simulink model "canrx_0x586"  (R2022b)
settings: Solver=VariableStepAuto  StartTime=0.0  StopTime=10.0  RelTol=1e-3
values from neighbouring files (symbols this model uses):
  K_CAN_GMLAN_RX_INVALID_SELECT = 0.0    [canrx_0x586.sldd]
  PLCANC_APCNTL_RQST_SEL_GMLAN = 1.0    [canrx_0x586.sldd]
  PLCANC_APCNTL_RQST_SEL_J1939 = 0.0    [canrx_0x586.sldd]
undefined symbols (not defined in the file or in its folder): K_CAN_GMLAN_RX_DEFAULT_GPS_ALTITUDE, K_CAN_GMLAN_RX_DEFAULT_GPS_ANTENNA_STAT, K_CAN_GMLAN_RX_DEFAULT_GPS_DIRECTION, K_CAN_GMLAN_RX_DEFAULT_GPS_HDOP, K_CAN_GMLAN_RX_DEFAULT_GPS_LATITUDE, K_CAN_GMLAN_RX_DEFAULT_GPS_LONGITUDE, K_CAN_GMLAN_RX_DEFAULT_GPS_SG_UB, K_CAN_GMLAN_RX_DEFAULT_GPS_TIME, K_CAN_GMLAN_RX_DEFAULT_GPS_VEH_SPEED, K_CAN_RQST_SEL_1, K_CAN_RQST_SEL_2, K_CAN_RX_SEL_2, K_RQST_DRCT_2
libraries: simulink x9
(part 1 of 2)
settings Model: DataDictionary=canrx_0x586.sldd  Creator=Castiel  LastModifiedBy=Castiel

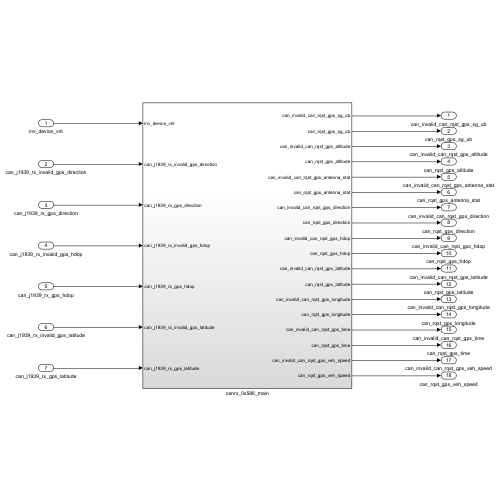
[thumbnail: Simulink's stored preview of the top-level diagram]
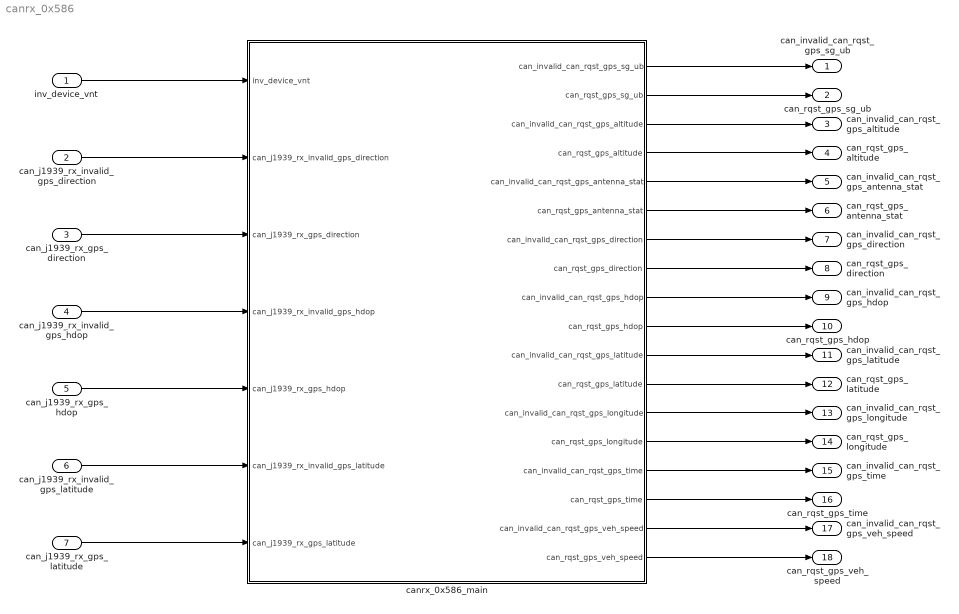
== system canrx_0x586 ==
  inv_device_vnt : Inport
  can_j1939_rx_invalid_gps_direction : Inport  Port=2
  can_j1939_rx_gps_direction : Inport  Port=3
  can_j1939_rx_invalid_gps_hdop : Inport  Port=4
  can_j1939_rx_gps_hdop : Inport  Port=5
  can_j1939_rx_invalid_gps_latitude : Inport  Port=6
  can_j1939_rx_gps_latitude : Inport  Port=7
  canrx_0x586_main : Subsystem
  can_invalid_can_rqst_gps_sg_ub : Outport
  can_rqst_gps_sg_ub : Outport  Port=2
  can_invalid_can_rqst_gps_altitude : Outport  Port=3
  can_rqst_gps_altitude : Outport  Port=4
  can_invalid_can_rqst_gps_antenna_stat : Outport  Port=5
  can_rqst_gps_antenna_stat : Outport  Port=6
  can_invalid_can_rqst_gps_direction : Outport  Port=7
  can_rqst_gps_direction : Outport  Port=8
  can_invalid_can_rqst_gps_hdop : Outport  Port=9
  can_rqst_gps_hdop : Outport  Port=10
  can_invalid_can_rqst_gps_latitude : Outport  Port=11
  can_rqst_gps_latitude : Outport  Port=12
  can_invalid_can_rqst_gps_longitude : Outport  Port=13
  can_rqst_gps_longitude : Outport  Port=14
  can_invalid_can_rqst_gps_time : Outport  Port=15
  can_rqst_gps_time : Outport  Port=16
  can_invalid_can_rqst_gps_veh_speed : Outport  Port=17
  can_rqst_gps_veh_speed : Outport  Port=18
  wires:
  inv_device_vnt/1 -> canrx_0x586_main/1(inv_device_vnt)
  can_j1939_rx_invalid_gps_direction/1 -> canrx_0x586_main/2(can_j1939_rx_invalid_gps_direction)
  can_j1939_rx_gps_direction/1 -> canrx_0x586_main/3(can_j1939_rx_gps_direction)
  can_j1939_rx_invalid_gps_hdop/1 -> canrx_0x586_main/4(can_j1939_rx_invalid_gps_hdop)
  can_j1939_rx_gps_hdop/1 -> canrx_0x586_main/5(can_j1939_rx_gps_hdop)
  can_j1939_rx_invalid_gps_latitude/1 -> canrx_0x586_main/6(can_j1939_rx_invalid_gps_latitude)
  can_j1939_rx_gps_latitude/1 -> canrx_0x586_main/7(can_j1939_rx_gps_latitude)
  canrx_0x586_main/1(can_invalid_can_rqst_gps_sg_ub) -> can_invalid_can_rqst_gps_sg_ub/1
  canrx_0x586_main/2(can_rqst_gps_sg_ub) -> can_rqst_gps_sg_ub/1
  canrx_0x586_main/3(can_invalid_can_rqst_gps_altitude) -> can_invalid_can_rqst_gps_altitude/1
  canrx_0x586_main/4(can_rqst_gps_altitude) -> can_rqst_gps_altitude/1
  canrx_0x586_main/5(can_invalid_can_rqst_gps_antenna_stat) -> can_invalid_can_rqst_gps_antenna_stat/1
  canrx_0x586_main/6(can_rqst_gps_antenna_stat) -> can_rqst_gps_antenna_stat/1
  canrx_0x586_main/7(can_invalid_can_rqst_gps_direction) -> can_invalid_can_rqst_gps_direction/1
  canrx_0x586_main/8(can_rqst_gps_direction) -> can_rqst_gps_direction/1
  canrx_0x586_main/9(can_invalid_can_rqst_gps_hdop) -> can_invalid_can_rqst_gps_hdop/1
  canrx_0x586_main/10(can_rqst_gps_hdop) -> can_rqst_gps_hdop/1
  canrx_0x586_main/11(can_invalid_can_rqst_gps_latitude) -> can_invalid_can_rqst_gps_latitude/1
  canrx_0x586_main/12(can_rqst_gps_latitude) -> can_rqst_gps_latitude/1
  canrx_0x586_main/13(can_invalid_can_rqst_gps_longitude) -> can_invalid_can_rqst_gps_longitude/1
  canrx_0x586_main/14(can_rqst_gps_longitude) -> can_rqst_gps_longitude/1
  canrx_0x586_main/15(can_invalid_can_rqst_gps_time) -> can_invalid_can_rqst_gps_time/1
  canrx_0x586_main/16(can_rqst_gps_time) -> can_rqst_gps_time/1
  canrx_0x586_main/17(can_invalid_can_rqst_gps_veh_speed) -> can_invalid_can_rqst_gps_veh_speed/1
  canrx_0x586_main/18(can_rqst_gps_veh_speed) -> can_rqst_gps_veh_speed/1

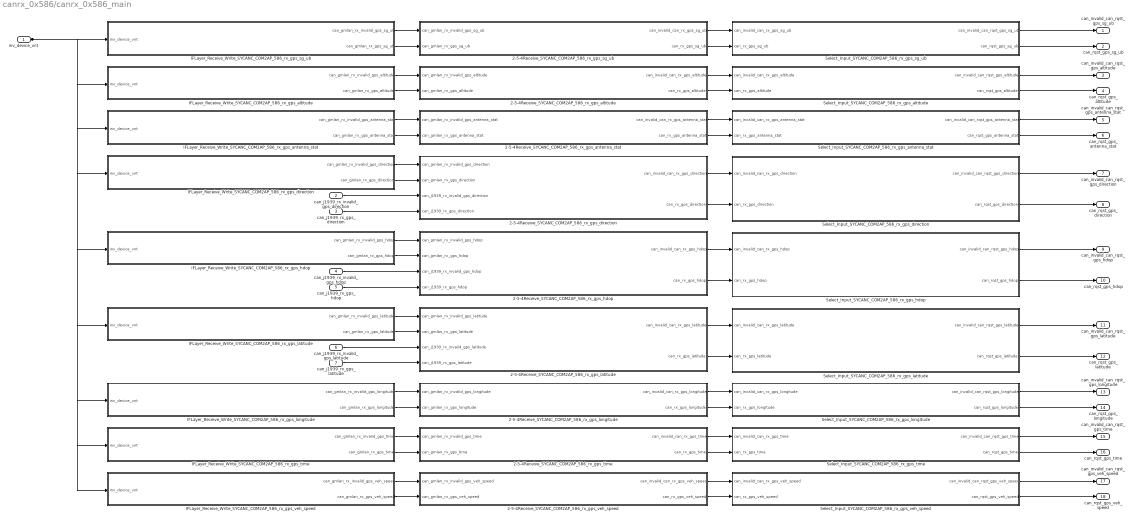
== system canrx_0x586/canrx_0x586_main ==
  inv_device_vnt : Inport
  can_j1939_rx_invalid_gps_direction : Inport  Port=2
  can_j1939_rx_gps_direction : Inport  Port=3
  can_j1939_rx_invalid_gps_hdop : Inport  Port=4
  can_j1939_rx_gps_hdop : Inport  Port=5
  can_j1939_rx_invalid_gps_latitude : Inport  Port=6
  can_j1939_rx_gps_latitude : Inport  Port=7
  2-5-4Receive_SYCANC_COM2AP_586_rx_gps_altitude : Subsystem  TreatAsAtomicUnit=on
      settings: RTWSystemCode=Nonreusable function
  2-5-4Receive_SYCANC_COM2AP_586_rx_gps_antenna_stat : Subsystem  TreatAsAtomicUnit=on
      settings: RTWSystemCode=Nonreusable function
  2-5-4Receive_SYCANC_COM2AP_586_rx_gps_direction : Subsystem  TreatAsAtomicUnit=on
      settings: RTWSystemCode=Nonreusable function
  2-5-4Receive_SYCANC_COM2AP_586_rx_gps_hdop : Subsystem  TreatAsAtomicUnit=on
      settings: RTWSystemCode=Nonreusable function
  2-5-4Receive_SYCANC_COM2AP_586_rx_gps_latitude : Subsystem  TreatAsAtomicUnit=on
      settings: RTWSystemCode=Nonreusable function
  2-5-4Receive_SYCANC_COM2AP_586_rx_gps_longitude : Subsystem  TreatAsAtomicUnit=on
      settings: RTWSystemCode=Nonreusable function
  2-5-4Receive_SYCANC_COM2AP_586_rx_gps_sg_ub : Subsystem  TreatAsAtomicUnit=on
      settings: RTWSystemCode=Nonreusable function
  2-5-4Receive_SYCANC_COM2AP_586_rx_gps_time : Subsystem  TreatAsAtomicUnit=on
      settings: RTWSystemCode=Nonreusable function
  2-5-4Receive_SYCANC_COM2AP_586_rx_gps_veh_speed : Subsystem  TreatAsAtomicUnit=on
      settings: RTWSystemCode=Nonreusable function
  IFLayer_Receive_Write_SYCANC_COM2AP_586_rx_gps_altitude : Subsystem  TreatAsAtomicUnit=on
      settings: RTWSystemCode=Nonreusable function
  IFLayer_Receive_Write_SYCANC_COM2AP_586_rx_gps_antenna_stat : Subsystem  TreatAsAtomicUnit=on
      settings: RTWSystemCode=Nonreusable function
  IFLayer_Receive_Write_SYCANC_COM2AP_586_rx_gps_direction : Subsystem  TreatAsAtomicUnit=on
      settings: RTWSystemCode=Nonreusable function
  IFLayer_Receive_Write_SYCANC_COM2AP_586_rx_gps_hdop : Subsystem  TreatAsAtomicUnit=on
      settings: RTWSystemCode=Nonreusable function
  IFLayer_Receive_Write_SYCANC_COM2AP_586_rx_gps_latitude : Subsystem  TreatAsAtomicUnit=on
      settings: RTWSystemCode=Nonreusable function
  IFLayer_Receive_Write_SYCANC_COM2AP_586_rx_gps_longitude : Subsystem  TreatAsAtomicUnit=on
      settings: RTWSystemCode=Nonreusable function
  IFLayer_Receive_Write_SYCANC_COM2AP_586_rx_gps_sg_ub : Subsystem  TreatAsAtomicUnit=on
      settings: RTWSystemCode=Nonreusable function
  IFLayer_Receive_Write_SYCANC_COM2AP_586_rx_gps_time : Subsystem  TreatAsAtomicUnit=on
      settings: RTWSystemCode=Nonreusable function
  IFLayer_Receive_Write_SYCANC_COM2AP_586_rx_gps_veh_speed : Subsystem  TreatAsAtomicUnit=on
      settings: RTWSystemCode=Nonreusable function
  Select_Input_SYCANC_COM2AP_586_rx_gps_altitude : Subsystem  TreatAsAtomicUnit=on
      settings: RTWSystemCode=Nonreusable function
  Select_Input_SYCANC_COM2AP_586_rx_gps_antenna_stat : Subsystem  TreatAsAtomicUnit=on
      settings: RTWSystemCode=Nonreusable function
  Select_Input_SYCANC_COM2AP_586_rx_gps_direction : Subsystem  TreatAsAtomicUnit=on
      settings: RTWSystemCode=Nonreusable function
  Select_Input_SYCANC_COM2AP_586_rx_gps_hdop : Subsystem  TreatAsAtomicUnit=on
      settings: RTWSystemCode=Nonreusable function
  Select_Input_SYCANC_COM2AP_586_rx_gps_latitude : Subsystem  TreatAsAtomicUnit=on
      settings: RTWSystemCode=Nonreusable function
  Select_Input_SYCANC_COM2AP_586_rx_gps_longitude : Subsystem  TreatAsAtomicUnit=on
      settings: RTWSystemCode=Nonreusable function
  Select_Input_SYCANC_COM2AP_586_rx_gps_sg_ub : Subsystem  TreatAsAtomicUnit=on
      settings: RTWSystemCode=Nonreusable function
  Select_Input_SYCANC_COM2AP_586_rx_gps_time : Subsystem  TreatAsAtomicUnit=on
      settings: RTWSystemCode=Nonreusable function
  Select_Input_SYCANC_COM2AP_586_rx_gps_veh_speed : Subsystem  TreatAsAtomicUnit=on
      settings: RTWSystemCode=Nonreusable function
  can_invalid_can_rqst_gps_sg_ub : Outport
  can_rqst_gps_sg_ub : Outport  Port=2
  can_invalid_can_rqst_gps_altitude : Outport  Port=3
  can_rqst_gps_altitude : Outport  Port=4
  can_invalid_can_rqst_gps_antenna_stat : Outport  Port=5
  can_rqst_gps_antenna_stat : Outport  Port=6
  can_invalid_can_rqst_gps_direction : Outport  Port=7
  can_rqst_gps_direction : Outport  Port=8
  can_invalid_can_rqst_gps_hdop : Outport  Port=9
  can_rqst_gps_hdop : Outport  Port=10
  can_invalid_can_rqst_gps_latitude : Outport  Port=11
  can_rqst_gps_latitude : Outport  Port=12
  can_invalid_can_rqst_gps_longitude : Outport  Port=13
  can_rqst_gps_longitude : Outport  Port=14
  can_invalid_can_rqst_gps_time : Outport  Port=15
  can_rqst_gps_time : Outport  Port=16
  can_invalid_can_rqst_gps_veh_speed : Outport  Port=17
  can_rqst_gps_veh_speed : Outport  Port=18
  wires:
  IFLayer_Receive_Write_SYCANC_COM2AP_586_rx_gps_sg_ub/2(can_gmlan_rx_gps_sg_ub) -> 2-5-4Receive_SYCANC_COM2AP_586_rx_gps_sg_ub/2(can_gmlan_rx_gps_sg_ub)
  IFLayer_Receive_Write_SYCANC_COM2AP_586_rx_gps_sg_ub/1(can_gmlan_rx_invalid_gps_sg_ub) -> 2-5-4Receive_SYCANC_COM2AP_586_rx_gps_sg_ub/1(can_gmlan_rx_invalid_gps_sg_ub)
  2-5-4Receive_SYCANC_COM2AP_586_rx_gps_sg_ub/1(can_invalid_can_rx_gps_sg_ub) -> Select_Input_SYCANC_COM2AP_586_rx_gps_sg_ub/1(can_invalid_can_rx_gps_sg_ub)
  2-5-4Receive_SYCANC_COM2AP_586_rx_gps_sg_ub/2(can_rx_gps_sg_ub) -> Select_Input_SYCANC_COM2AP_586_rx_gps_sg_ub/2(can_rx_gps_sg_ub)
  inv_device_vnt/1 -> IFLayer_Receive_Write_SYCANC_COM2AP_586_rx_gps_sg_ub/1(inv_device_vnt), IFLayer_Receive_Write_SYCANC_COM2AP_586_rx_gps_altitude/1(inv_device_vnt), IFLayer_Receive_Write_SYCANC_COM2AP_586_rx_gps_antenna_stat/1(inv_device_vnt), IFLayer_Receive_Write_SYCANC_COM2AP_586_rx_gps_direction/1(inv_device_vnt), IFLayer_Receive_Write_SYCANC_COM2AP_586_rx_gps_hdop/1(inv_device_vnt), IFLayer_Receive_Write_SYCANC_COM2AP_586_rx_gps_latitude/1(inv_device_vnt), IFLayer_Receive_Write_SYCANC_COM2AP_586_rx_gps_longitude/1(inv_device_vnt), IFLayer_Receive_Write_SYCANC_COM2AP_586_rx_gps_time/1(inv_device_vnt), IFLayer_Receive_Write_SYCANC_COM2AP_586_rx_gps_veh_speed/1(inv_device_vnt)
  Select_Input_SYCANC_COM2AP_586_rx_gps_sg_ub/1(can_invalid_can_rqst_gps_sg_ub) -> can_invalid_can_rqst_gps_sg_ub/1
  Select_Input_SYCANC_COM2AP_586_rx_gps_sg_ub/2(can_rqst_gps_sg_ub) -> can_rqst_gps_sg_ub/1
  IFLayer_Receive_Write_SYCANC_COM2AP_586_rx_gps_altitude/2(can_gmlan_rx_gps_altitude) -> 2-5-4Receive_SYCANC_COM2AP_586_rx_gps_altitude/2(can_gmlan_rx_gps_altitude)
  IFLayer_Receive_Write_SYCANC_COM2AP_586_rx_gps_altitude/1(can_gmlan_rx_invalid_gps_altitude) -> 2-5-4Receive_SYCANC_COM2AP_586_rx_gps_altitude/1(can_gmlan_rx_invalid_gps_altitude)
  2-5-4Receive_SYCANC_COM2AP_586_rx_gps_altitude/1(can_invalid_can_rx_gps_altitude) -> Select_Input_SYCANC_COM2AP_586_rx_gps_altitude/1(can_invalid_can_rx_gps_altitude)
  2-5-4Receive_SYCANC_COM2AP_586_rx_gps_altitude/2(can_rx_gps_altitude) -> Select_Input_SYCANC_COM2AP_586_rx_gps_altitude/2(can_rx_gps_altitude)
  Select_Input_SYCANC_COM2AP_586_rx_gps_altitude/1(can_invalid_can_rqst_gps_altitude) -> can_invalid_can_rqst_gps_altitude/1
  Select_Input_SYCANC_COM2AP_586_rx_gps_altitude/2(can_rqst_gps_altitude) -> can_rqst_gps_altitude/1
  IFLayer_Receive_Write_SYCANC_COM2AP_586_rx_gps_antenna_stat/2(can_gmlan_rx_gps_antenna_stat) -> 2-5-4Receive_SYCANC_COM2AP_586_rx_gps_antenna_stat/2(can_gmlan_rx_gps_antenna_stat)
  IFLayer_Receive_Write_SYCANC_COM2AP_586_rx_gps_antenna_stat/1(can_gmlan_rx_invalid_gps_antenna_stat) -> 2-5-4Receive_SYCANC_COM2AP_586_rx_gps_antenna_stat/1(can_gmlan_rx_invalid_gps_antenna_stat)
  2-5-4Receive_SYCANC_COM2AP_586_rx_gps_antenna_stat/1(can_invalid_can_rx_gps_antenna_stat) -> Select_Input_SYCANC_COM2AP_586_rx_gps_antenna_stat/1(can_invalid_can_rx_gps_antenna_stat)
  2-5-4Receive_SYCANC_COM2AP_586_rx_gps_antenna_stat/2(can_rx_gps_antenna_stat) -> Select_Input_SYCANC_COM2AP_586_rx_gps_antenna_stat/2(can_rx_gps_antenna_stat)
  Select_Input_SYCANC_COM2AP_586_rx_gps_antenna_stat/1(can_invalid_can_rqst_gps_antenna_stat) -> can_invalid_can_rqst_gps_antenna_stat/1
  Select_Input_SYCANC_COM2AP_586_rx_gps_antenna_stat/2(can_rqst_gps_antenna_stat) -> can_rqst_gps_antenna_stat/1
  IFLayer_Receive_Write_SYCANC_COM2AP_586_rx_gps_direction/2(can_gmlan_rx_gps_direction) -> 2-5-4Receive_SYCANC_COM2AP_586_rx_gps_direction/2(can_gmlan_rx_gps_direction)
  IFLayer_Receive_Write_SYCANC_COM2AP_586_rx_gps_direction/1(can_gmlan_rx_invalid_gps_direction) -> 2-5-4Receive_SYCANC_COM2AP_586_rx_gps_direction/1(can_gmlan_rx_invalid_gps_direction)
  2-5-4Receive_SYCANC_COM2AP_586_rx_gps_direction/1(can_invalid_can_rx_gps_direction) -> Select_Input_SYCANC_COM2AP_586_rx_gps_direction/1(can_invalid_can_rx_gps_direction)
  2-5-4Receive_SYCANC_COM2AP_586_rx_gps_direction/2(can_rx_gps_direction) -> Select_Input_SYCANC_COM2AP_586_rx_gps_direction/2(can_rx_gps_direction)
  can_j1939_rx_invalid_gps_direction/1 -> 2-5-4Receive_SYCANC_COM2AP_586_rx_gps_direction/3(can_j1939_rx_invalid_gps_direction)
  can_j1939_rx_gps_direction/1 -> 2-5-4Receive_SYCANC_COM2AP_586_rx_gps_direction/4(can_j1939_rx_gps_direction)
  Select_Input_SYCANC_COM2AP_586_rx_gps_direction/1(can_invalid_can_rqst_gps_direction) -> can_invalid_can_rqst_gps_direction/1
  Select_Input_SYCANC_COM2AP_586_rx_gps_direction/2(can_rqst_gps_direction) -> can_rqst_gps_direction/1
  IFLayer_Receive_Write_SYCANC_COM2AP_586_rx_gps_hdop/2(can_gmlan_rx_gps_hdop) -> 2-5-4Receive_SYCANC_COM2AP_586_rx_gps_hdop/2(can_gmlan_rx_gps_hdop)
  IFLayer_Receive_Write_SYCANC_COM2AP_586_rx_gps_hdop/1(can_gmlan_rx_invalid_gps_hdop) -> 2-5-4Receive_SYCANC_COM2AP_586_rx_gps_hdop/1(can_gmlan_rx_invalid_gps_hdop)
  2-5-4Receive_SYCANC_COM2AP_586_rx_gps_hdop/1(can_invalid_can_rx_gps_hdop) -> Select_Input_SYCANC_COM2AP_586_rx_gps_hdop/1(can_invalid_can_rx_gps_hdop)
  2-5-4Receive_SYCANC_COM2AP_586_rx_gps_hdop/2(can_rx_gps_hdop) -> Select_Input_SYCANC_COM2AP_586_rx_gps_hdop/2(can_rx_gps_hdop)
  can_j1939_rx_invalid_gps_hdop/1 -> 2-5-4Receive_SYCANC_COM2AP_586_rx_gps_hdop/3(can_j1939_rx_invalid_gps_hdop)
  can_j1939_rx_gps_hdop/1 -> 2-5-4Receive_SYCANC_COM2AP_586_rx_gps_hdop/4(can_j1939_rx_gps_hdop)
  Select_Input_SYCANC_COM2AP_586_rx_gps_hdop/1(can_invalid_can_rqst_gps_hdop) -> can_invalid_can_rqst_gps_hdop/1
  Select_Input_SYCANC_COM2AP_586_rx_gps_hdop/2(can_rqst_gps_hdop) -> can_rqst_gps_hdop/1
  IFLayer_Receive_Write_SYCANC_COM2AP_586_rx_gps_latitude/2(can_gmlan_rx_gps_latitude) -> 2-5-4Receive_SYCANC_COM2AP_586_rx_gps_latitude/2(can_gmlan_rx_gps_latitude)
  IFLayer_Receive_Write_SYCANC_COM2AP_586_rx_gps_latitude/1(can_gmlan_rx_invalid_gps_latitude) -> 2-5-4Receive_SYCANC_COM2AP_586_rx_gps_latitude/1(can_gmlan_rx_invalid_gps_latitude)
  2-5-4Receive_SYCANC_COM2AP_586_rx_gps_latitude/1(can_invalid_can_rx_gps_latitude) -> Select_Input_SYCANC_COM2AP_586_rx_gps_latitude/1(can_invalid_can_rx_gps_latitude)
  2-5-4Receive_SYCANC_COM2AP_586_rx_gps_latitude/2(can_rx_gps_latitude) -> Select_Input_SYCANC_COM2AP_586_rx_gps_latitude/2(can_rx_gps_latitude)
  can_j1939_rx_invalid_gps_latitude/1 -> 2-5-4Receive_SYCANC_COM2AP_586_rx_gps_latitude/3(can_j1939_rx_invalid_gps_latitude)
  can_j1939_rx_gps_latitude/1 -> 2-5-4Receive_SYCANC_COM2AP_586_rx_gps_latitude/4(can_j1939_rx_gps_latitude)
  Select_Input_SYCANC_COM2AP_586_rx_gps_latitude/1(can_invalid_can_rqst_gps_latitude) -> can_invalid_can_rqst_gps_latitude/1
  Select_Input_SYCANC_COM2AP_586_rx_gps_latitude/2(can_rqst_gps_latitude) -> can_rqst_gps_latitude/1
  IFLayer_Receive_Write_SYCANC_COM2AP_586_rx_gps_longitude/2(can_gmlan_rx_gps_longitude) -> 2-5-4Receive_SYCANC_COM2AP_586_rx_gps_longitude/2(can_gmlan_rx_gps_longitude)
  IFLayer_Receive_Write_SYCANC_COM2AP_586_rx_gps_longitude/1(can_gmlan_rx_invalid_gps_longitude) -> 2-5-4Receive_SYCANC_COM2AP_586_rx_gps_longitude/1(can_gmlan_rx_invalid_gps_longitude)
  2-5-4Receive_SYCANC_COM2AP_586_rx_gps_longitude/1(can_invalid_can_rx_gps_longitude) -> Select_Input_SYCANC_COM2AP_586_rx_gps_longitude/1(can_invalid_can_rx_gps_longitude)
  2-5-4Receive_SYCANC_COM2AP_586_rx_gps_longitude/2(can_rx_gps_longitude) -> Select_Input_SYCANC_COM2AP_586_rx_gps_longitude/2(can_rx_gps_longitude)
  Select_Input_SYCANC_COM2AP_586_rx_gps_longitude/1(can_invalid_can_rqst_gps_longitude) -> can_invalid_can_rqst_gps_longitude/1
  Select_Input_SYCANC_COM2AP_586_rx_gps_longitude/2(can_rqst_gps_longitude) -> can_rqst_gps_longitude/1
  IFLayer_Receive_Write_SYCANC_COM2AP_586_rx_gps_time/2(can_gmlan_rx_gps_time) -> 2-5-4Receive_SYCANC_COM2AP_586_rx_gps_time/2(can_gmlan_rx_gps_time)
  IFLayer_Receive_Write_SYCANC_COM2AP_586_rx_gps_time/1(can_gmlan_rx_invalid_gps_time) -> 2-5-4Receive_SYCANC_COM2AP_586_rx_gps_time/1(can_gmlan_rx_invalid_gps_time)
  2-5-4Receive_SYCANC_COM2AP_586_rx_gps_time/1(can_invalid_can_rx_gps_time) -> Select_Input_SYCANC_COM2AP_586_rx_gps_time/1(can_invalid_can_rx_gps_time)
  2-5-4Receive_SYCANC_COM2AP_586_rx_gps_time/2(can_rx_gps_time) -> Select_Input_SYCANC_COM2AP_586_rx_gps_time/2(can_rx_gps_time)
  Select_Input_SYCANC_COM2AP_586_rx_gps_time/1(can_invalid_can_rqst_gps_time) -> can_invalid_can_rqst_gps_time/1
  Select_Input_SYCANC_COM2AP_586_rx_gps_time/2(can_rqst_gps_time) -> can_rqst_gps_time/1
  IFLayer_Receive_Write_SYCANC_COM2AP_586_rx_gps_veh_speed/2(can_gmlan_rx_gps_veh_speed) -> 2-5-4Receive_SYCANC_COM2AP_586_rx_gps_veh_speed/2(can_gmlan_rx_gps_veh_speed)
  IFLayer_Receive_Write_SYCANC_COM2AP_586_rx_gps_veh_speed/1(can_gmlan_rx_invalid_gps_veh_speed) -> 2-5-4Receive_SYCANC_COM2AP_586_rx_gps_veh_speed/1(can_gmlan_rx_invalid_gps_veh_speed)
  2-5-4Receive_SYCANC_COM2AP_586_rx_gps_veh_speed/1(can_invalid_can_rx_gps_veh_speed) -> Select_Input_SYCANC_COM2AP_586_rx_gps_veh_speed/1(can_invalid_can_rx_gps_veh_speed)
  2-5-4Receive_SYCANC_COM2AP_586_rx_gps_veh_speed/2(can_rx_gps_veh_speed) -> Select_Input_SYCANC_COM2AP_586_rx_gps_veh_speed/2(can_rx_gps_veh_speed)
  Select_Input_SYCANC_COM2AP_586_rx_gps_veh_speed/1(can_invalid_can_rqst_gps_veh_speed) -> can_invalid_can_rqst_gps_veh_speed/1
  Select_Input_SYCANC_COM2AP_586_rx_gps_veh_speed/2(can_rqst_gps_veh_speed) -> can_rqst_gps_veh_speed/1

== system canrx_0x586/canrx_0x586_main/2-5-4Receive_SYCANC_COM2AP_586_rx_gps_altitude ==
  can_gmlan_rx_invalid_gps_altitude : Inport
  can_gmlan_rx_gps_altitude : Inport  Port=2
  can_invalid_can_rx_gps_altitude : Outport
  can_rx_gps_altitude : Outport  Port=2
  wires:
  can_gmlan_rx_gps_altitude/1 -> can_rx_gps_altitude/1
  can_gmlan_rx_invalid_gps_altitude/1 -> can_invalid_can_rx_gps_altitude/1

== system canrx_0x586/canrx_0x586_main/2-5-4Receive_SYCANC_COM2AP_586_rx_gps_antenna_stat ==
  can_gmlan_rx_invalid_gps_antenna_stat : Inport
  can_gmlan_rx_gps_antenna_stat : Inport  Port=2
  can_invalid_can_rx_gps_antenna_stat : Outport
  can_rx_gps_antenna_stat : Outport  Port=2
  wires:
  can_gmlan_rx_gps_antenna_stat/1 -> can_rx_gps_antenna_stat/1
  can_gmlan_rx_invalid_gps_antenna_stat/1 -> can_invalid_can_rx_gps_antenna_stat/1

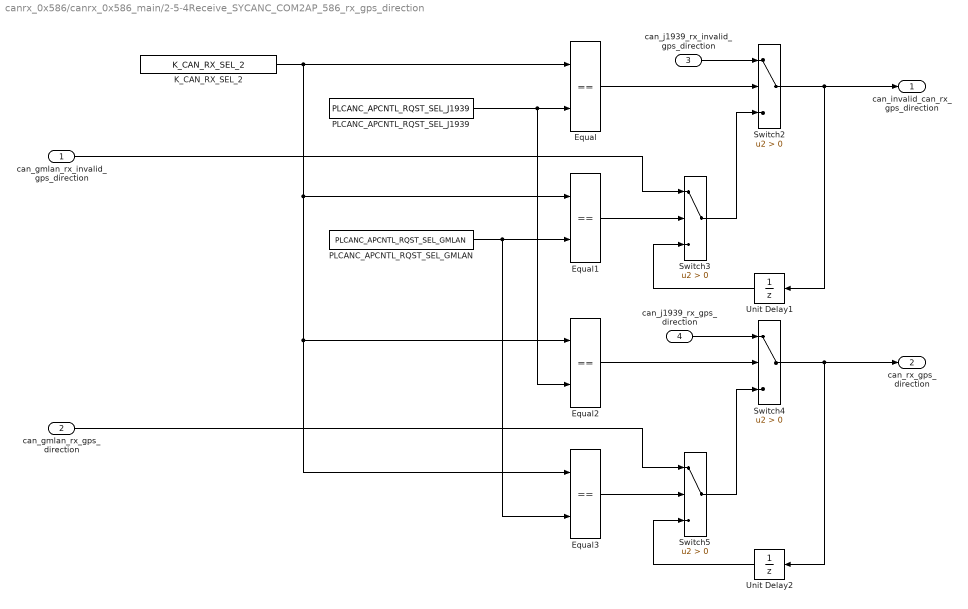
== system canrx_0x586/canrx_0x586_main/2-5-4Receive_SYCANC_COM2AP_586_rx_gps_direction ==
  can_gmlan_rx_invalid_gps_direction : Inport
  can_gmlan_rx_gps_direction : Inport  Port=2
  can_j1939_rx_invalid_gps_direction : Inport  Port=3
  can_j1939_rx_gps_direction : Inport  Port=4
  Equal{,1..3} (4 alike) : RelationalOperator  Operator===  OutDataTypeStr=boolean  RndMeth=Simplest  InputSameDT=off
  K_CAN_RX_SEL_2 : Constant  Value=K_CAN_RX_SEL_2
  PLCANC_APCNTL_RQST_SEL_GMLAN : Constant  Value=PLCANC_APCNTL_RQST_SEL_GMLAN
  PLCANC_APCNTL_RQST_SEL_J1939 : Constant  Value=PLCANC_APCNTL_RQST_SEL_J1939
  Switch{2..5} (4 alike) : Switch  Criteria=u2 > Threshold  SaturateOnIntegerOverflow=off  InputSameDT=off
  Unit Delay1 : UnitDelay  SampleTime=-1  HasFrameUpgradeWarning=on
  Unit Delay2 : UnitDelay  SampleTime=-1  HasFrameUpgradeWarning=on
  can_invalid_can_rx_gps_direction : Outport
  can_rx_gps_direction : Outport  Port=2
  wires:
  Switch3/1 -> Switch2/3
  can_j1939_rx_gps_direction/1 -> Switch4/1
  K_CAN_RX_SEL_2/1 -> Equal/1, Equal1/1, Equal2/1, Equal3/1
  Switch4/1 -> can_rx_gps_direction/1, Unit Delay2/1
  PLCANC_APCNTL_RQST_SEL_J1939/1 -> Equal/2, Equal2/2
  can_gmlan_rx_gps_direction/1 -> Switch5/1
  Equal2/1 -> Switch4/2
  can_j1939_rx_invalid_gps_direction/1 -> Switch2/1
  PLCANC_APCNTL_RQST_SEL_GMLAN/1 -> Equal1/2, Equal3/2
  can_gmlan_rx_invalid_gps_direction/1 -> Switch3/1
  Switch5/1 -> Switch4/3
  Equal3/1 -> Switch5/2
  Equal1/1 -> Switch3/2
  Unit Delay2/1 -> Switch5/3
  Switch2/1 -> can_invalid_can_rx_gps_direction/1, Unit Delay1/1
  Unit Delay1/1 -> Switch3/3
  Equal/1 -> Switch2/2

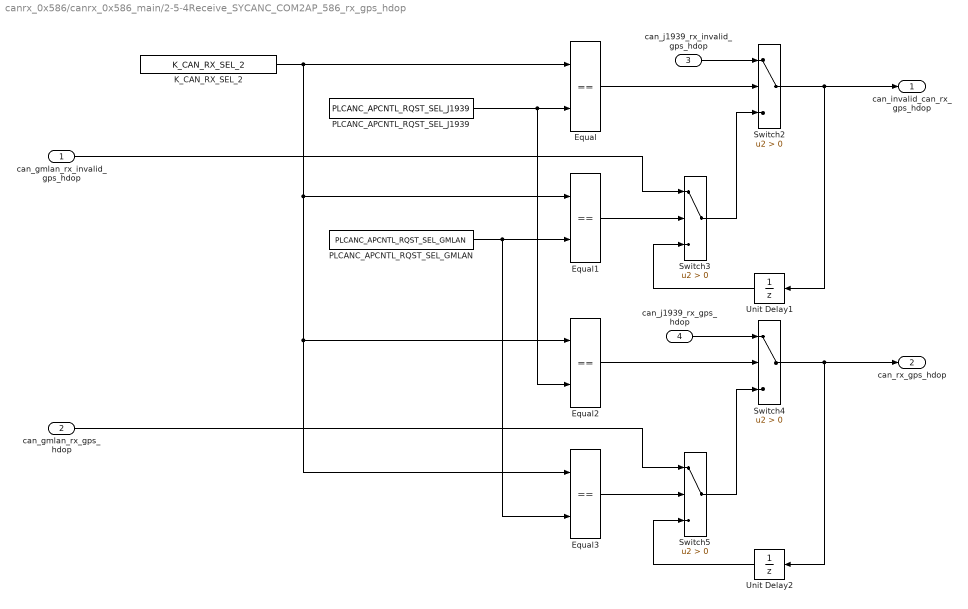
== system canrx_0x586/canrx_0x586_main/2-5-4Receive_SYCANC_COM2AP_586_rx_gps_hdop ==
  can_gmlan_rx_invalid_gps_hdop : Inport
  can_gmlan_rx_gps_hdop : Inport  Port=2
  can_j1939_rx_invalid_gps_hdop : Inport  Port=3
  can_j1939_rx_gps_hdop : Inport  Port=4
  Equal{,1..3} (4 alike) : RelationalOperator  Operator===  OutDataTypeStr=boolean  RndMeth=Simplest  InputSameDT=off
  K_CAN_RX_SEL_2 : Constant  Value=K_CAN_RX_SEL_2
  PLCANC_APCNTL_RQST_SEL_GMLAN : Constant  Value=PLCANC_APCNTL_RQST_SEL_GMLAN
  PLCANC_APCNTL_RQST_SEL_J1939 : Constant  Value=PLCANC_APCNTL_RQST_SEL_J1939
  Switch{2..5} (4 alike) : Switch  Criteria=u2 > Threshold  SaturateOnIntegerOverflow=off  InputSameDT=off
  Unit Delay1 : UnitDelay  SampleTime=-1  HasFrameUpgradeWarning=on
  Unit Delay2 : UnitDelay  SampleTime=-1  HasFrameUpgradeWarning=on
  can_invalid_can_rx_gps_hdop : Outport
  can_rx_gps_hdop : Outport  Port=2
  wires:
  Switch3/1 -> Switch2/3
  can_j1939_rx_gps_hdop/1 -> Switch4/1
  K_CAN_RX_SEL_2/1 -> Equal/1, Equal1/1, Equal2/1, Equal3/1
  Switch4/1 -> can_rx_gps_hdop/1, Unit Delay2/1
  PLCANC_APCNTL_RQST_SEL_J1939/1 -> Equal/2, Equal2/2
  can_gmlan_rx_gps_hdop/1 -> Switch5/1
  Equal2/1 -> Switch4/2
  can_j1939_rx_invalid_gps_hdop/1 -> Switch2/1
  PLCANC_APCNTL_RQST_SEL_GMLAN/1 -> Equal1/2, Equal3/2
  can_gmlan_rx_invalid_gps_hdop/1 -> Switch3/1
  Switch5/1 -> Switch4/3
  Equal3/1 -> Switch5/2
  Equal1/1 -> Switch3/2
  Unit Delay2/1 -> Switch5/3
  Switch2/1 -> can_invalid_can_rx_gps_hdop/1, Unit Delay1/1
  Unit Delay1/1 -> Switch3/3
  Equal/1 -> Switch2/2

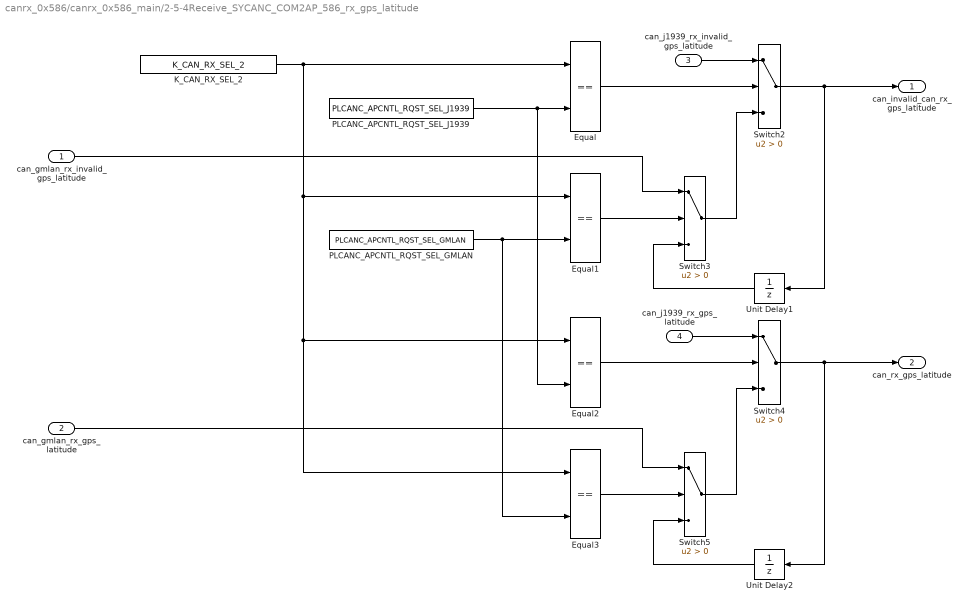
== system canrx_0x586/canrx_0x586_main/2-5-4Receive_SYCANC_COM2AP_586_rx_gps_latitude ==
  can_gmlan_rx_invalid_gps_latitude : Inport
  can_gmlan_rx_gps_latitude : Inport  Port=2
  can_j1939_rx_invalid_gps_latitude : Inport  Port=3
  can_j1939_rx_gps_latitude : Inport  Port=4
  Equal{,1..3} (4 alike) : RelationalOperator  Operator===  OutDataTypeStr=boolean  RndMeth=Simplest  InputSameDT=off
  K_CAN_RX_SEL_2 : Constant  Value=K_CAN_RX_SEL_2
  PLCANC_APCNTL_RQST_SEL_GMLAN : Constant  Value=PLCANC_APCNTL_RQST_SEL_GMLAN
  PLCANC_APCNTL_RQST_SEL_J1939 : Constant  Value=PLCANC_APCNTL_RQST_SEL_J1939
  Switch{2..5} (4 alike) : Switch  Criteria=u2 > Threshold  SaturateOnIntegerOverflow=off  InputSameDT=off
  Unit Delay1 : UnitDelay  SampleTime=-1  HasFrameUpgradeWarning=on
  Unit Delay2 : UnitDelay  SampleTime=-1  HasFrameUpgradeWarning=on
  can_invalid_can_rx_gps_latitude : Outport
  can_rx_gps_latitude : Outport  Port=2
  wires:
  Switch3/1 -> Switch2/3
  can_j1939_rx_gps_latitude/1 -> Switch4/1
  K_CAN_RX_SEL_2/1 -> Equal/1, Equal1/1, Equal2/1, Equal3/1
  Switch4/1 -> can_rx_gps_latitude/1, Unit Delay2/1
  PLCANC_APCNTL_RQST_SEL_J1939/1 -> Equal/2, Equal2/2
  can_gmlan_rx_gps_latitude/1 -> Switch5/1
  Equal2/1 -> Switch4/2
  can_j1939_rx_invalid_gps_latitude/1 -> Switch2/1
  PLCANC_APCNTL_RQST_SEL_GMLAN/1 -> Equal1/2, Equal3/2
  can_gmlan_rx_invalid_gps_latitude/1 -> Switch3/1
  Switch5/1 -> Switch4/3
  Equal3/1 -> Switch5/2
  Equal1/1 -> Switch3/2
  Unit Delay2/1 -> Switch5/3
  Switch2/1 -> can_invalid_can_rx_gps_latitude/1, Unit Delay1/1
  Unit Delay1/1 -> Switch3/3
  Equal/1 -> Switch2/2

== system canrx_0x586/canrx_0x586_main/2-5-4Receive_SYCANC_COM2AP_586_rx_gps_longitude ==
  can_gmlan_rx_invalid_gps_longitude : Inport
  can_gmlan_rx_gps_longitude : Inport  Port=2
  can_invalid_can_rx_gps_longitude : Outport
  can_rx_gps_longitude : Outport  Port=2
  wires:
  can_gmlan_rx_gps_longitude/1 -> can_rx_gps_longitude/1
  can_gmlan_rx_invalid_gps_longitude/1 -> can_invalid_can_rx_gps_longitude/1

== system canrx_0x586/canrx_0x586_main/2-5-4Receive_SYCANC_COM2AP_586_rx_gps_sg_ub ==
  can_gmlan_rx_invalid_gps_sg_ub : Inport
  can_gmlan_rx_gps_sg_ub : Inport  Port=2
  can_invalid_can_rx_gps_sg_ub : Outport
  can_rx_gps_sg_ub : Outport  Port=2
  wires:
  can_gmlan_rx_gps_sg_ub/1 -> can_rx_gps_sg_ub/1
  can_gmlan_rx_invalid_gps_sg_ub/1 -> can_invalid_can_rx_gps_sg_ub/1

== system canrx_0x586/canrx_0x586_main/2-5-4Receive_SYCANC_COM2AP_586_rx_gps_time ==
  can_gmlan_rx_invalid_gps_time : Inport
  can_gmlan_rx_gps_time : Inport  Port=2
  can_invalid_can_rx_gps_time : Outport
  can_rx_gps_time : Outport  Port=2
  wires:
  can_gmlan_rx_gps_time/1 -> can_rx_gps_time/1
  can_gmlan_rx_invalid_gps_time/1 -> can_invalid_can_rx_gps_time/1

== system canrx_0x586/canrx_0x586_main/2-5-4Receive_SYCANC_COM2AP_586_rx_gps_veh_speed ==
  can_gmlan_rx_invalid_gps_veh_speed : Inport
  can_gmlan_rx_gps_veh_speed : Inport  Port=2
  can_invalid_can_rx_gps_veh_speed : Outport
  can_rx_gps_veh_speed : Outport  Port=2
  wires:
  can_gmlan_rx_gps_veh_speed/1 -> can_rx_gps_veh_speed/1
  can_gmlan_rx_invalid_gps_veh_speed/1 -> can_invalid_can_rx_gps_veh_speed/1

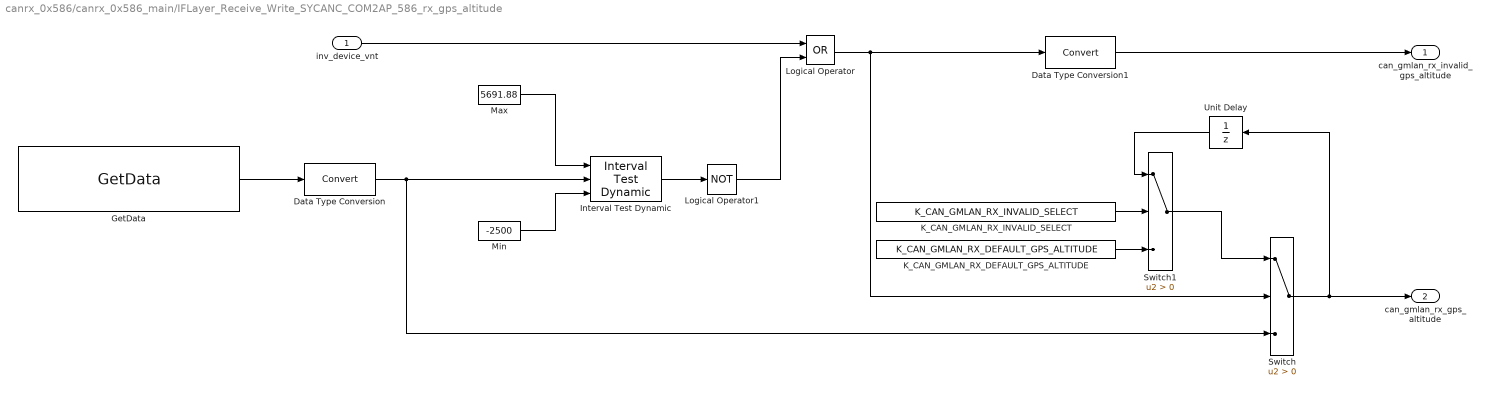
== system canrx_0x586/canrx_0x586_main/IFLayer_Receive_Write_SYCANC_COM2AP_586_rx_gps_altitude ==
  inv_device_vnt : Inport
  Data Type Conversion : DataTypeConversion  ConvertRealWorld=Stored Integer (SI)  SaturateOnIntegerOverflow=off  RndMeth=Floor
  Data Type Conversion1 : DataTypeConversion  ConvertRealWorld=Stored Integer (SI)  SaturateOnIntegerOverflow=off  RndMeth=Floor
  GetData : S-Function  FunctionName=GetData  Parameters=interface,signalType  SFunctionDeploymentMode=off  EnableBusSupport=off  mask{interface=SYCANC_COM2AP_586_rx_gps_altitude, signalType=SW}
      mask prompts: signalType "Signal Type"
      mask TypeOptions signalType: UB | SB | UW | SW | UD | SD
      mask DialogControl Container4 Prompt: Singal Parameter
      mask Display:
      | interfaceName = get_param(gcbh, "interface");
      | s = strcat(interfaceName);
      | disp(s);
  Interval Test Dynamic : simulink/Logic and Bit Operations/Interval Test Dynamic  IntervalClosedRight=on  IntervalClosedLeft=on  OutDataTypeStr=boolean
  K_CAN_GMLAN_RX_DEFAULT_GPS_ALTITUDE : Constant  Value=K_CAN_GMLAN_RX_DEFAULT_GPS_ALTITUDE  OutDataTypeStr=Inherit: Inherit via back propagation
  K_CAN_GMLAN_RX_INVALID_SELECT : Constant  Value=K_CAN_GMLAN_RX_INVALID_SELECT  OutDataTypeStr=Inherit: Inherit via back propagation
  Logical Operator : Logic  Operator=OR  AllPortsSameDT=off  OutDataTypeStr=boolean
  Logical Operator1 : Logic  Operator=NOT  AllPortsSameDT=off  OutDataTypeStr=boolean
  Max : Constant  Value=5691.88  OutDataTypeStr=Inherit: Inherit via back propagation
  Min : Constant  Value=-2500  OutDataTypeStr=Inherit: Inherit via back propagation
  Switch : Switch  Criteria=u2 > Threshold  SaturateOnIntegerOverflow=off  InputSameDT=off
  Switch1 : Switch  Criteria=u2 > Threshold  SaturateOnIntegerOverflow=off  InputSameDT=off
  Unit Delay : UnitDelay  SampleTime=-1  HasFrameUpgradeWarning=on
  can_gmlan_rx_invalid_gps_altitude : Outport
  can_gmlan_rx_gps_altitude : Outport  Port=2
  wires:
  inv_device_vnt/1 -> Logical Operator/1
  K_CAN_GMLAN_RX_INVALID_SELECT/1 -> Switch1/2
  Data Type Conversion1/1 -> can_gmlan_rx_invalid_gps_altitude/1
  Logical Operator/1 -> Data Type Conversion1/1, Switch/2
  K_CAN_GMLAN_RX_DEFAULT_GPS_ALTITUDE/1 -> Switch1/3
  Switch1/1 -> Switch/1
  Switch/1 -> can_gmlan_rx_gps_altitude/1, Unit Delay/1
  Logical Operator1/1 -> Logical Operator/2
  Max/1 -> Interval Test Dynamic/1
  Min/1 -> Interval Test Dynamic/3
  Unit Delay/1 -> Switch1/1
  GetData/1 -> Data Type Conversion/1
  Interval Test Dynamic/1 -> Logical Operator1/1
  Data Type Conversion/1 -> Switch/3, Interval Test Dynamic/2

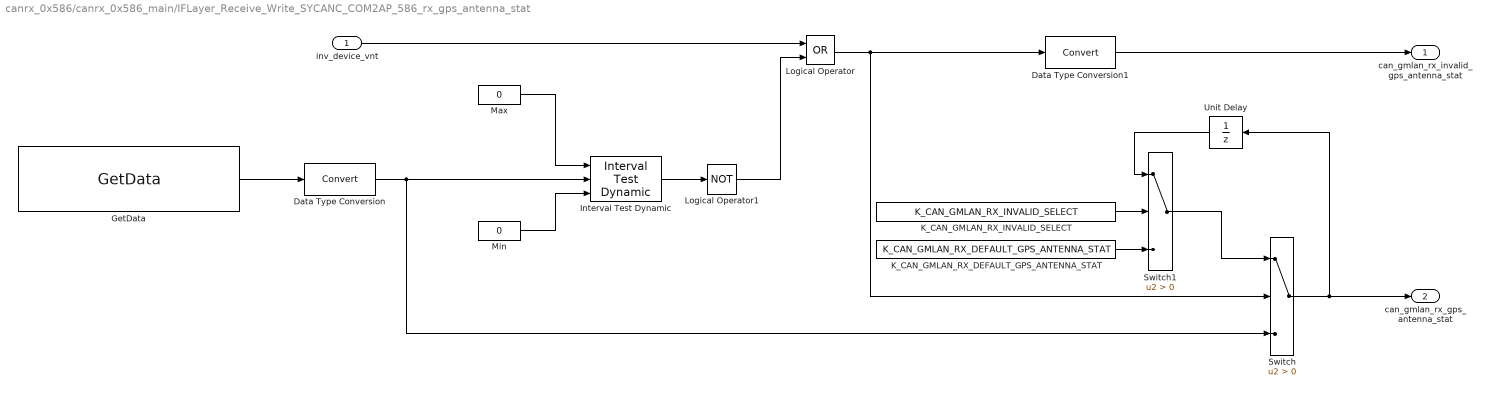
== system canrx_0x586/canrx_0x586_main/IFLayer_Receive_Write_SYCANC_COM2AP_586_rx_gps_antenna_stat ==
  inv_device_vnt : Inport
  Data Type Conversion : DataTypeConversion  ConvertRealWorld=Stored Integer (SI)  SaturateOnIntegerOverflow=off  RndMeth=Floor
  Data Type Conversion1 : DataTypeConversion  ConvertRealWorld=Stored Integer (SI)  SaturateOnIntegerOverflow=off  RndMeth=Floor
  GetData : S-Function  FunctionName=GetData  Parameters=interface,signalType  SFunctionDeploymentMode=off  EnableBusSupport=off  mask{interface=SYCANC_COM2AP_586_rx_gps_antenna_stat, signalType=UW}
      mask prompts: signalType "Signal Type"
      mask TypeOptions signalType: UB | SB | UW | SW | UD | SD
      mask DialogControl Container4 Prompt: Singal Parameter
      mask Display:
      | interfaceName = get_param(gcbh, "interface");
      | s = strcat(interfaceName);
      | disp(s);
  Interval Test Dynamic : simulink/Logic and Bit Operations/Interval Test Dynamic  IntervalClosedRight=on  IntervalClosedLeft=on  OutDataTypeStr=boolean
  K_CAN_GMLAN_RX_DEFAULT_GPS_ANTENNA_STAT : Constant  Value=K_CAN_GMLAN_RX_DEFAULT_GPS_ANTENNA_STAT  OutDataTypeStr=Inherit: Inherit via back propagation
  K_CAN_GMLAN_RX_INVALID_SELECT : Constant  Value=K_CAN_GMLAN_RX_INVALID_SELECT  OutDataTypeStr=Inherit: Inherit via back propagation
  Logical Operator : Logic  Operator=OR  AllPortsSameDT=off  OutDataTypeStr=boolean
  Logical Operator1 : Logic  Operator=NOT  AllPortsSameDT=off  OutDataTypeStr=boolean
  Max : Constant  Value=0  OutDataTypeStr=Inherit: Inherit via back propagation
  Min : Constant  Value=0  OutDataTypeStr=Inherit: Inherit via back propagation
  Switch : Switch  Criteria=u2 > Threshold  SaturateOnIntegerOverflow=off  InputSameDT=off
  Switch1 : Switch  Criteria=u2 > Threshold  SaturateOnIntegerOverflow=off  InputSameDT=off
  Unit Delay : UnitDelay  SampleTime=-1  HasFrameUpgradeWarning=on
  can_gmlan_rx_invalid_gps_antenna_stat : Outport
  can_gmlan_rx_gps_antenna_stat : Outport  Port=2
  wires:
  inv_device_vnt/1 -> Logical Operator/1
  K_CAN_GMLAN_RX_INVALID_SELECT/1 -> Switch1/2
  Data Type Conversion1/1 -> can_gmlan_rx_invalid_gps_antenna_stat/1
  Logical Operator/1 -> Data Type Conversion1/1, Switch/2
  K_CAN_GMLAN_RX_DEFAULT_GPS_ANTENNA_STAT/1 -> Switch1/3
  Switch1/1 -> Switch/1
  Switch/1 -> can_gmlan_rx_gps_antenna_stat/1, Unit Delay/1
  Logical Operator1/1 -> Logical Operator/2
  Max/1 -> Interval Test Dynamic/1
  Min/1 -> Interval Test Dynamic/3
  Unit Delay/1 -> Switch1/1
  GetData/1 -> Data Type Conversion/1
  Interval Test Dynamic/1 -> Logical Operator1/1
  Data Type Conversion/1 -> Switch/3, Interval Test Dynamic/2

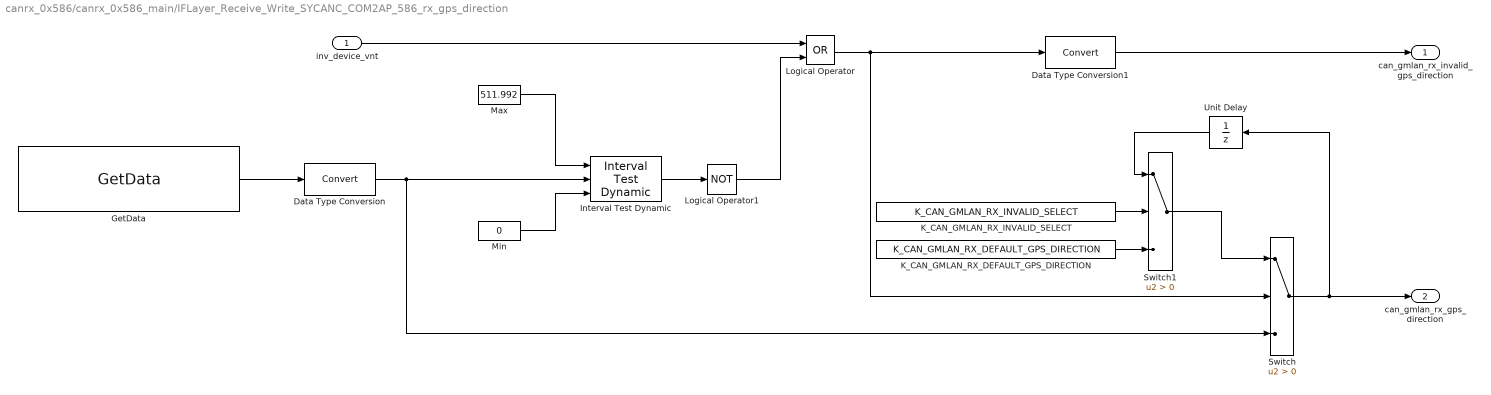
== system canrx_0x586/canrx_0x586_main/IFLayer_Receive_Write_SYCANC_COM2AP_586_rx_gps_direction ==
  inv_device_vnt : Inport
  Data Type Conversion : DataTypeConversion  ConvertRealWorld=Stored Integer (SI)  SaturateOnIntegerOverflow=off  RndMeth=Floor
  Data Type Conversion1 : DataTypeConversion  ConvertRealWorld=Stored Integer (SI)  SaturateOnIntegerOverflow=off  RndMeth=Floor
  GetData : S-Function  FunctionName=GetData  Parameters=interface,signalType  SFunctionDeploymentMode=off  EnableBusSupport=off  mask{interface=SYCANC_COM2AP_586_rx_gps_direction, signalType=UD}
      mask prompts: signalType "Signal Type"
      mask TypeOptions signalType: UB | SB | UW | SW | UD | SD
      mask DialogControl Container4 Prompt: Singal Parameter
      mask Display:
      | interfaceName = get_param(gcbh, "interface");
      | s = strcat(interfaceName);
      | disp(s);
  Interval Test Dynamic : simulink/Logic and Bit Operations/Interval Test Dynamic  IntervalClosedRight=on  IntervalClosedLeft=on  OutDataTypeStr=boolean
  K_CAN_GMLAN_RX_DEFAULT_GPS_DIRECTION : Constant  Value=K_CAN_GMLAN_RX_DEFAULT_GPS_DIRECTION  OutDataTypeStr=Inherit: Inherit via back propagation
  K_CAN_GMLAN_RX_INVALID_SELECT : Constant  Value=K_CAN_GMLAN_RX_INVALID_SELECT  OutDataTypeStr=Inherit: Inherit via back propagation
  Logical Operator : Logic  Operator=OR  AllPortsSameDT=off  OutDataTypeStr=boolean
  Logical Operator1 : Logic  Operator=NOT  AllPortsSameDT=off  OutDataTypeStr=boolean
  Max : Constant  Value=511.992  OutDataTypeStr=Inherit: Inherit via back propagation
  Min : Constant  Value=0  OutDataTypeStr=Inherit: Inherit via back propagation
  Switch : Switch  Criteria=u2 > Threshold  SaturateOnIntegerOverflow=off  InputSameDT=off
  Switch1 : Switch  Criteria=u2 > Threshold  SaturateOnIntegerOverflow=off  InputSameDT=off
  Unit Delay : UnitDelay  SampleTime=-1  HasFrameUpgradeWarning=on
  can_gmlan_rx_invalid_gps_direction : Outport
  can_gmlan_rx_gps_direction : Outport  Port=2
  wires:
  inv_device_vnt/1 -> Logical Operator/1
  K_CAN_GMLAN_RX_INVALID_SELECT/1 -> Switch1/2
  Data Type Conversion1/1 -> can_gmlan_rx_invalid_gps_direction/1
  Logical Operator/1 -> Data Type Conversion1/1, Switch/2
  K_CAN_GMLAN_RX_DEFAULT_GPS_DIRECTION/1 -> Switch1/3
  Switch1/1 -> Switch/1
  Switch/1 -> can_gmlan_rx_gps_direction/1, Unit Delay/1
  Logical Operator1/1 -> Logical Operator/2
  Max/1 -> Interval Test Dynamic/1
  Min/1 -> Interval Test Dynamic/3
  Unit Delay/1 -> Switch1/1
  GetData/1 -> Data Type Conversion/1
  Interval Test Dynamic/1 -> Logical Operator1/1
  Data Type Conversion/1 -> Switch/3, Interval Test Dynamic/2

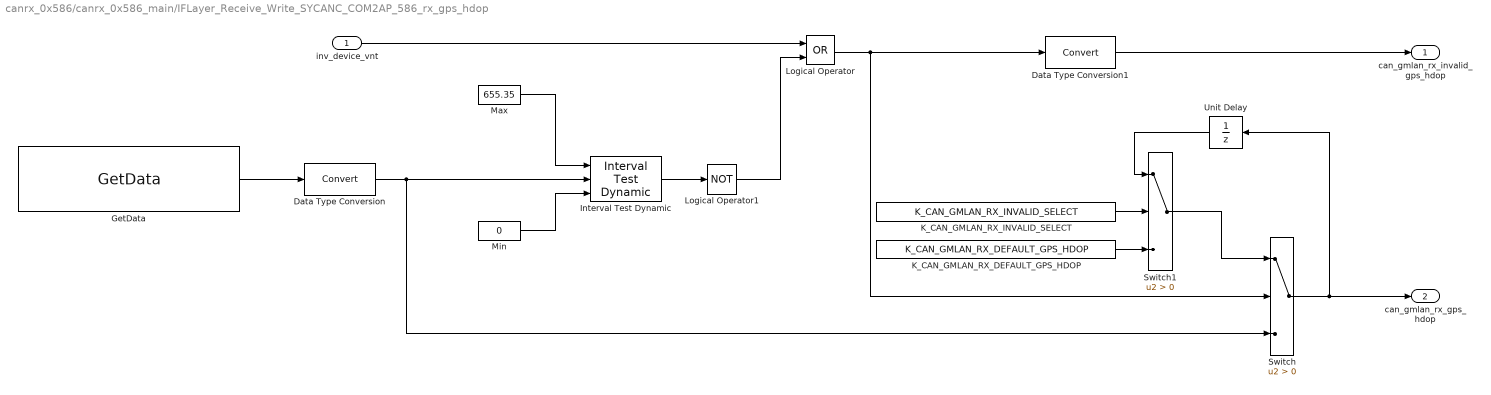
== system canrx_0x586/canrx_0x586_main/IFLayer_Receive_Write_SYCANC_COM2AP_586_rx_gps_hdop ==
  inv_device_vnt : Inport
  Data Type Conversion : DataTypeConversion  ConvertRealWorld=Stored Integer (SI)  SaturateOnIntegerOverflow=off  RndMeth=Floor
  Data Type Conversion1 : DataTypeConversion  ConvertRealWorld=Stored Integer (SI)  SaturateOnIntegerOverflow=off  RndMeth=Floor
  GetData : S-Function  FunctionName=GetData  Parameters=interface,signalType  SFunctionDeploymentMode=off  EnableBusSupport=off  mask{interface=SYCANC_COM2AP_586_rx_gps_hdop, signalType=UW}
      mask prompts: signalType "Signal Type"
      mask TypeOptions signalType: UB | SB | UW | SW | UD | SD
      mask DialogControl Container4 Prompt: Singal Parameter
      mask Display:
      | interfaceName = get_param(gcbh, "interface");
      | s = strcat(interfaceName);
      | disp(s);
  Interval Test Dynamic : simulink/Logic and Bit Operations/Interval Test Dynamic  IntervalClosedRight=on  IntervalClosedLeft=on  OutDataTypeStr=boolean
  K_CAN_GMLAN_RX_DEFAULT_GPS_HDOP : Constant  Value=K_CAN_GMLAN_RX_DEFAULT_GPS_HDOP  OutDataTypeStr=Inherit: Inherit via back propagation
  K_CAN_GMLAN_RX_INVALID_SELECT : Constant  Value=K_CAN_GMLAN_RX_INVALID_SELECT  OutDataTypeStr=Inherit: Inherit via back propagation
  Logical Operator : Logic  Operator=OR  AllPortsSameDT=off  OutDataTypeStr=boolean
  Logical Operator1 : Logic  Operator=NOT  AllPortsSameDT=off  OutDataTypeStr=boolean
  Max : Constant  Value=655.35  OutDataTypeStr=Inherit: Inherit via back propagation
  Min : Constant  Value=0  OutDataTypeStr=Inherit: Inherit via back propagation
  Switch : Switch  Criteria=u2 > Threshold  SaturateOnIntegerOverflow=off  InputSameDT=off
  Switch1 : Switch  Criteria=u2 > Threshold  SaturateOnIntegerOverflow=off  InputSameDT=off
  Unit Delay : UnitDelay  SampleTime=-1  HasFrameUpgradeWarning=on
  can_gmlan_rx_invalid_gps_hdop : Outport
  can_gmlan_rx_gps_hdop : Outport  Port=2
  wires:
  inv_device_vnt/1 -> Logical Operator/1
  K_CAN_GMLAN_RX_INVALID_SELECT/1 -> Switch1/2
  Data Type Conversion1/1 -> can_gmlan_rx_invalid_gps_hdop/1
  Logical Operator/1 -> Data Type Conversion1/1, Switch/2
  K_CAN_GMLAN_RX_DEFAULT_GPS_HDOP/1 -> Switch1/3
  Switch1/1 -> Switch/1
  Switch/1 -> can_gmlan_rx_gps_hdop/1, Unit Delay/1
  Logical Operator1/1 -> Logical Operator/2
  Max/1 -> Interval Test Dynamic/1
  Min/1 -> Interval Test Dynamic/3
  Unit Delay/1 -> Switch1/1
  GetData/1 -> Data Type Conversion/1
  Interval Test Dynamic/1 -> Logical Operator1/1
  Data Type Conversion/1 -> Switch/3, Interval Test Dynamic/2

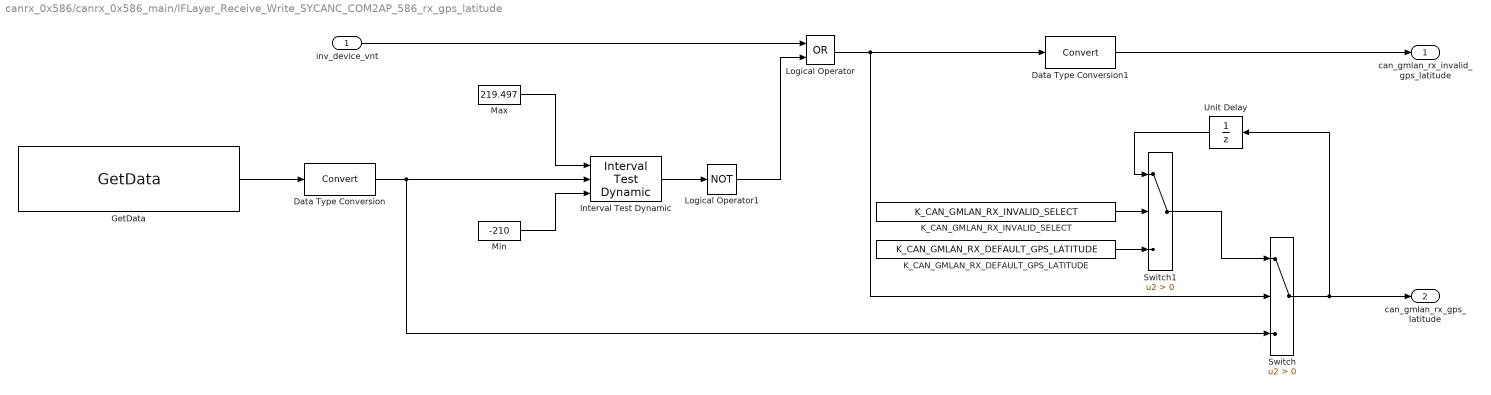
== system canrx_0x586/canrx_0x586_main/IFLayer_Receive_Write_SYCANC_COM2AP_586_rx_gps_latitude ==
  inv_device_vnt : Inport
  Data Type Conversion : DataTypeConversion  ConvertRealWorld=Stored Integer (SI)  SaturateOnIntegerOverflow=off  RndMeth=Floor
  Data Type Conversion1 : DataTypeConversion  ConvertRealWorld=Stored Integer (SI)  SaturateOnIntegerOverflow=off  RndMeth=Floor
  GetData : S-Function  FunctionName=GetData  Parameters=interface,signalType  SFunctionDeploymentMode=off  EnableBusSupport=off  mask{interface=SYCANC_COM2AP_586_rx_gps_latitude, signalType=SD}
      mask prompts: signalType "Signal Type"
      mask TypeOptions signalType: UB | SB | UW | SW | UD | SD
      mask DialogControl Container4 Prompt: Singal Parameter
      mask Display:
      | interfaceName = get_param(gcbh, "interface");
      | s = strcat(interfaceName);
      | disp(s);
  Interval Test Dynamic : simulink/Logic and Bit Operations/Interval Test Dynamic  IntervalClosedRight=on  IntervalClosedLeft=on  OutDataTypeStr=boolean
  K_CAN_GMLAN_RX_DEFAULT_GPS_LATITUDE : Constant  Value=K_CAN_GMLAN_RX_DEFAULT_GPS_LATITUDE  OutDataTypeStr=Inherit: Inherit via back propagation
  K_CAN_GMLAN_RX_INVALID_SELECT : Constant  Value=K_CAN_GMLAN_RX_INVALID_SELECT  OutDataTypeStr=Inherit: Inherit via back propagation
  Logical Operator : Logic  Operator=OR  AllPortsSameDT=off  OutDataTypeStr=boolean
  Logical Operator1 : Logic  Operator=NOT  AllPortsSameDT=off  OutDataTypeStr=boolean
  Max : Constant  Value=219.497  OutDataTypeStr=Inherit: Inherit via back propagation
  Min : Constant  Value=-210  OutDataTypeStr=Inherit: Inherit via back propagation
  Switch : Switch  Criteria=u2 > Threshold  SaturateOnIntegerOverflow=off  InputSameDT=off
  Switch1 : Switch  Criteria=u2 > Threshold  SaturateOnIntegerOverflow=off  InputSameDT=off
  Unit Delay : UnitDelay  SampleTime=-1  HasFrameUpgradeWarning=on
  can_gmlan_rx_invalid_gps_latitude : Outport
  can_gmlan_rx_gps_latitude : Outport  Port=2
  wires:
  inv_device_vnt/1 -> Logical Operator/1
  K_CAN_GMLAN_RX_INVALID_SELECT/1 -> Switch1/2
  Data Type Conversion1/1 -> can_gmlan_rx_invalid_gps_latitude/1
  Logical Operator/1 -> Data Type Conversion1/1, Switch/2
  K_CAN_GMLAN_RX_DEFAULT_GPS_LATITUDE/1 -> Switch1/3
  Switch1/1 -> Switch/1
  Switch/1 -> can_gmlan_rx_gps_latitude/1, Unit Delay/1
  Logical Operator1/1 -> Logical Operator/2
  Max/1 -> Interval Test Dynamic/1
  Min/1 -> Interval Test Dynamic/3
  Unit Delay/1 -> Switch1/1
  GetData/1 -> Data Type Conversion/1
  Interval Test Dynamic/1 -> Logical Operator1/1
  Data Type Conversion/1 -> Switch/3, Interval Test Dynamic/2

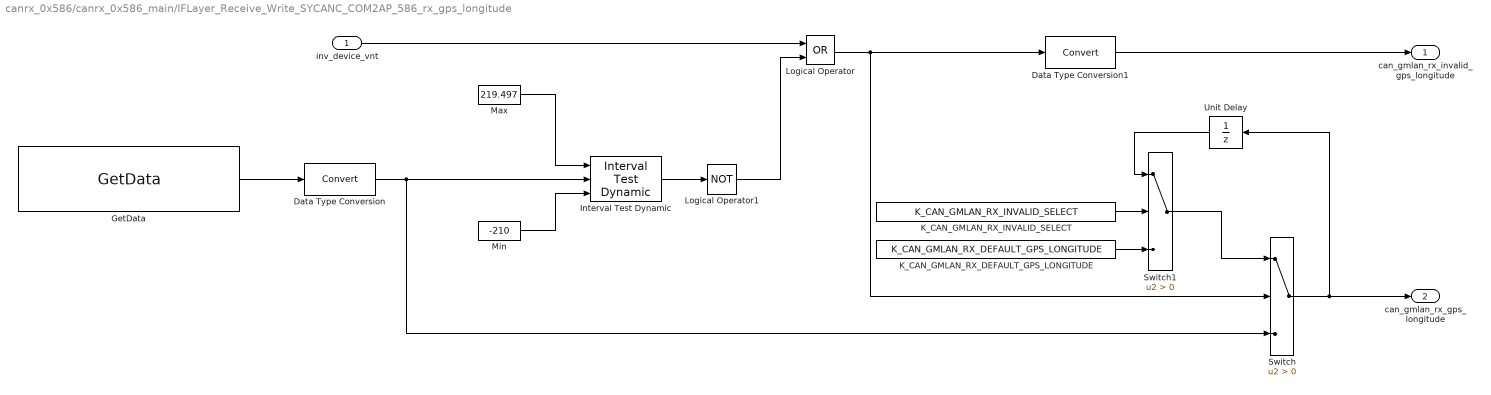
== system canrx_0x586/canrx_0x586_main/IFLayer_Receive_Write_SYCANC_COM2AP_586_rx_gps_longitude ==
  inv_device_vnt : Inport
  Data Type Conversion : DataTypeConversion  ConvertRealWorld=Stored Integer (SI)  SaturateOnIntegerOverflow=off  RndMeth=Floor
  Data Type Conversion1 : DataTypeConversion  ConvertRealWorld=Stored Integer (SI)  SaturateOnIntegerOverflow=off  RndMeth=Floor
  GetData : S-Function  FunctionName=GetData  Parameters=interface,signalType  SFunctionDeploymentMode=off  EnableBusSupport=off  mask{interface=SYCANC_COM2AP_586_rx_gps_longitude, signalType=SD}
      mask prompts: signalType "Signal Type"
      mask TypeOptions signalType: UB | SB | UW | SW | UD | SD
      mask DialogControl Container4 Prompt: Singal Parameter
      mask Display:
      | interfaceName = get_param(gcbh, "interface");
      | s = strcat(interfaceName);
      | disp(s);
  Interval Test Dynamic : simulink/Logic and Bit Operations/Interval Test Dynamic  IntervalClosedRight=on  IntervalClosedLeft=on  OutDataTypeStr=boolean
  K_CAN_GMLAN_RX_DEFAULT_GPS_LONGITUDE : Constant  Value=K_CAN_GMLAN_RX_DEFAULT_GPS_LONGITUDE  OutDataTypeStr=Inherit: Inherit via back propagation
  K_CAN_GMLAN_RX_INVALID_SELECT : Constant  Value=K_CAN_GMLAN_RX_INVALID_SELECT  OutDataTypeStr=Inherit: Inherit via back propagation
  Logical Operator : Logic  Operator=OR  AllPortsSameDT=off  OutDataTypeStr=boolean
  Logical Operator1 : Logic  Operator=NOT  AllPortsSameDT=off  OutDataTypeStr=boolean
  Max : Constant  Value=219.497  OutDataTypeStr=Inherit: Inherit via back propagation
  Min : Constant  Value=-210  OutDataTypeStr=Inherit: Inherit via back propagation
  Switch : Switch  Criteria=u2 > Threshold  SaturateOnIntegerOverflow=off  InputSameDT=off
  Switch1 : Switch  Criteria=u2 > Threshold  SaturateOnIntegerOverflow=off  InputSameDT=off
  Unit Delay : UnitDelay  SampleTime=-1  HasFrameUpgradeWarning=on
  can_gmlan_rx_invalid_gps_longitude : Outport
  can_gmlan_rx_gps_longitude : Outport  Port=2
  wires:
  inv_device_vnt/1 -> Logical Operator/1
  K_CAN_GMLAN_RX_INVALID_SELECT/1 -> Switch1/2
  Data Type Conversion1/1 -> can_gmlan_rx_invalid_gps_longitude/1
  Logical Operator/1 -> Data Type Conversion1/1, Switch/2
  K_CAN_GMLAN_RX_DEFAULT_GPS_LONGITUDE/1 -> Switch1/3
  Switch1/1 -> Switch/1
  Switch/1 -> can_gmlan_rx_gps_longitude/1, Unit Delay/1
  Logical Operator1/1 -> Logical Operator/2
  Max/1 -> Interval Test Dynamic/1
  Min/1 -> Interval Test Dynamic/3
  Unit Delay/1 -> Switch1/1
  GetData/1 -> Data Type Conversion/1
  Interval Test Dynamic/1 -> Logical Operator1/1
  Data Type Conversion/1 -> Switch/3, Interval Test Dynamic/2

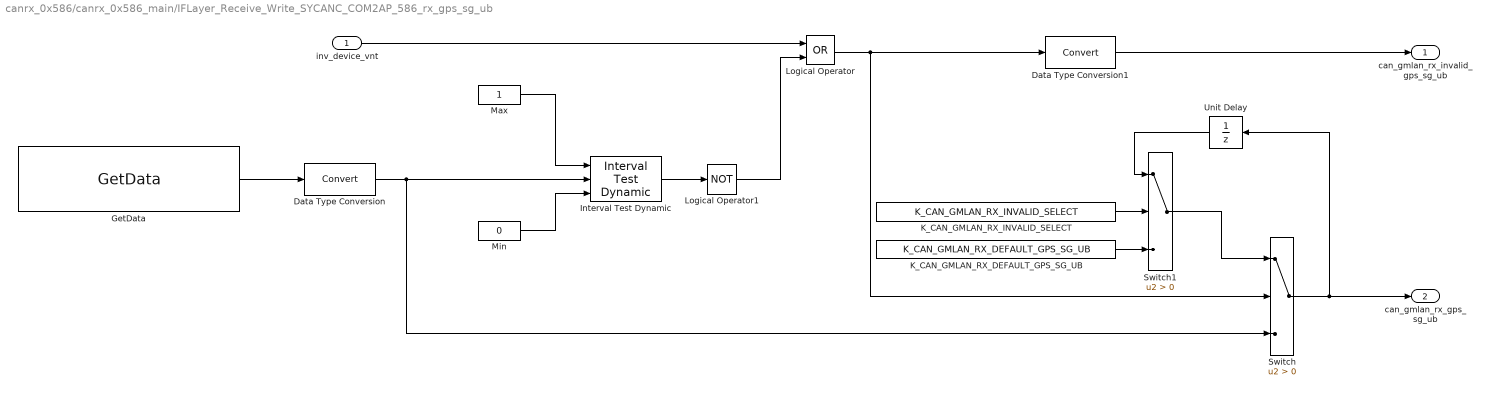
== system canrx_0x586/canrx_0x586_main/IFLayer_Receive_Write_SYCANC_COM2AP_586_rx_gps_sg_ub ==
  inv_device_vnt : Inport
  Data Type Conversion : DataTypeConversion  ConvertRealWorld=Stored Integer (SI)  SaturateOnIntegerOverflow=off  RndMeth=Floor
  Data Type Conversion1 : DataTypeConversion  ConvertRealWorld=Stored Integer (SI)  SaturateOnIntegerOverflow=off  RndMeth=Floor
  GetData : S-Function  FunctionName=GetData  Parameters=interface,signalType  SFunctionDeploymentMode=off  EnableBusSupport=off  mask{interface=SYCANC_COM2AP_586_rx_gps_sg_ub, signalType=UB}
      mask prompts: signalType "Signal Type"
      mask TypeOptions signalType: UB | SB | UW | SW | UD | SD
      mask DialogControl Container4 Prompt: Singal Parameter
      mask Display:
      | interfaceName = get_param(gcbh, "interface");
      | s = strcat(interfaceName);
      | disp(s);
  Interval Test Dynamic : simulink/Logic and Bit Operations/Interval Test Dynamic  IntervalClosedRight=on  IntervalClosedLeft=on  OutDataTypeStr=boolean
  K_CAN_GMLAN_RX_DEFAULT_GPS_SG_UB : Constant  Value=K_CAN_GMLAN_RX_DEFAULT_GPS_SG_UB  OutDataTypeStr=Inherit: Inherit via back propagation
  K_CAN_GMLAN_RX_INVALID_SELECT : Constant  Value=K_CAN_GMLAN_RX_INVALID_SELECT  OutDataTypeStr=Inherit: Inherit via back propagation
  Logical Operator : Logic  Operator=OR  AllPortsSameDT=off  OutDataTypeStr=boolean
  Logical Operator1 : Logic  Operator=NOT  AllPortsSameDT=off  OutDataTypeStr=boolean
  Max : Constant  OutDataTypeStr=Inherit: Inherit via back propagation
  Min : Constant  Value=0  OutDataTypeStr=Inherit: Inherit via back propagation
  Switch : Switch  Criteria=u2 > Threshold  SaturateOnIntegerOverflow=off  InputSameDT=off
  Switch1 : Switch  Criteria=u2 > Threshold  SaturateOnIntegerOverflow=off  InputSameDT=off
  Unit Delay : UnitDelay  SampleTime=-1  HasFrameUpgradeWarning=on
  can_gmlan_rx_invalid_gps_sg_ub : Outport
  can_gmlan_rx_gps_sg_ub : Outport  Port=2
  wires:
  inv_device_vnt/1 -> Logical Operator/1
  K_CAN_GMLAN_RX_INVALID_SELECT/1 -> Switch1/2
  Data Type Conversion1/1 -> can_gmlan_rx_invalid_gps_sg_ub/1
  Logical Operator/1 -> Data Type Conversion1/1, Switch/2
  K_CAN_GMLAN_RX_DEFAULT_GPS_SG_UB/1 -> Switch1/3
  Switch1/1 -> Switch/1
  Switch/1 -> can_gmlan_rx_gps_sg_ub/1, Unit Delay/1
  Logical Operator1/1 -> Logical Operator/2
  Max/1 -> Interval Test Dynamic/1
  Min/1 -> Interval Test Dynamic/3
  Unit Delay/1 -> Switch1/1
  GetData/1 -> Data Type Conversion/1
  Interval Test Dynamic/1 -> Logical Operator1/1
  Data Type Conversion/1 -> Switch/3, Interval Test Dynamic/2

== system canrx_0x586/canrx_0x586_main/IFLayer_Receive_Write_SYCANC_COM2AP_586_rx_gps_time ==
  inv_device_vnt : Inport
  Data Type Conversion : DataTypeConversion  ConvertRealWorld=Stored Integer (SI)  SaturateOnIntegerOverflow=off  RndMeth=Floor
  Data Type Conversion1 : DataTypeConversion  ConvertRealWorld=Stored Integer (SI)  SaturateOnIntegerOverflow=off  RndMeth=Floor
  GetData : S-Function  FunctionName=GetData  Parameters=interface,signalType  SFunctionDeploymentMode=off  EnableBusSupport=off  mask{interface=SYCANC_COM2AP_586_rx_gps_time, signalType=UB}
      mask prompts: signalType "Signal Type"
      mask TypeOptions signalType: UB | SB | UW | SW | UD | SD
      mask DialogControl Container4 Prompt: Singal Parameter
      mask Display:
      | interfaceName = get_param(gcbh, "interface");
      | s = strcat(interfaceName);
      | disp(s);
  Interval Test Dynamic : simulink/Logic and Bit Operations/Interval Test Dynamic  IntervalClosedRight=on  IntervalClosedLeft=on  OutDataTypeStr=boolean
  K_CAN_GMLAN_RX_DEFAULT_GPS_TIME : Constant  Value=K_CAN_GMLAN_RX_DEFAULT_GPS_TIME  OutDataTypeStr=Inherit: Inherit via back propagation
  K_CAN_GMLAN_RX_INVALID_SELECT : Constant  Value=K_CAN_GMLAN_RX_INVALID_SELECT  OutDataTypeStr=Inherit: Inherit via back propagation
  Logical Operator : Logic  Operator=OR  AllPortsSameDT=off  OutDataTypeStr=boolean
  Logical Operator1 : Logic  Operator=NOT  AllPortsSameDT=off  OutDataTypeStr=boolean
  Max : Constant  Value=4294970000  OutDataTypeStr=Inherit: Inherit via back propagation
  Min : Constant  Value=0  OutDataTypeStr=Inherit: Inherit via back propagation
  Switch : Switch  Criteria=u2 > Threshold  SaturateOnIntegerOverflow=off  InputSameDT=off
  Switch1 : Switch  Criteria=u2 > Threshold  SaturateOnIntegerOverflow=off  InputSameDT=off
  Unit Delay : UnitDelay  SampleTime=-1  HasFrameUpgradeWarning=on
  can_gmlan_rx_invalid_gps_time : Outport
  can_gmlan_rx_gps_time : Outport  Port=2
  wires:
  inv_device_vnt/1 -> Logical Operator/1
  K_CAN_GMLAN_RX_INVALID_SELECT/1 -> Switch1/2
  Data Type Conversion1/1 -> can_gmlan_rx_invalid_gps_time/1
  Logical Operator/1 -> Data Type Conversion1/1, Switch/2
  K_CAN_GMLAN_RX_DEFAULT_GPS_TIME/1 -> Switch1/3
  Switch1/1 -> Switch/1
  Switch/1 -> can_gmlan_rx_gps_time/1, Unit Delay/1
  Logical Operator1/1 -> Logical Operator/2
  Max/1 -> Interval Test Dynamic/1
  Min/1 -> Interval Test Dynamic/3
  Unit Delay/1 -> Switch1/1
  GetData/1 -> Data Type Conversion/1
  Interval Test Dynamic/1 -> Logical Operator1/1
  Data Type Conversion/1 -> Switch/3, Interval Test Dynamic/2

== system canrx_0x586/canrx_0x586_main/IFLayer_Receive_Write_SYCANC_COM2AP_586_rx_gps_veh_speed ==
  inv_device_vnt : Inport
  Data Type Conversion : DataTypeConversion  ConvertRealWorld=Stored Integer (SI)  SaturateOnIntegerOverflow=off  RndMeth=Floor
  Data Type Conversion1 : DataTypeConversion  ConvertRealWorld=Stored Integer (SI)  SaturateOnIntegerOverflow=off  RndMeth=Floor
  GetData : S-Function  FunctionName=GetData  Parameters=interface,signalType  SFunctionDeploymentMode=off  EnableBusSupport=off  mask{interface=SYCANC_COM2AP_586_rx_gps_veh_speed, signalType=UW}
      mask prompts: signalType "Signal Type"
      mask TypeOptions signalType: UB | SB | UW | SW | UD | SD
      mask DialogControl Container4 Prompt: Singal Parameter
      mask Display:
      | interfaceName = get_param(gcbh, "interface");
      | s = strcat(interfaceName);
      | disp(s);
  Interval Test Dynamic : simulink/Logic and Bit Operations/Interval Test Dynamic  IntervalClosedRight=on  IntervalClosedLeft=on  OutDataTypeStr=boolean
  K_CAN_GMLAN_RX_DEFAULT_GPS_VEH_SPEED : Constant  Value=K_CAN_GMLAN_RX_DEFAULT_GPS_VEH_SPEED  OutDataTypeStr=Inherit: Inherit via back propagation
  K_CAN_GMLAN_RX_INVALID_SELECT : Constant  Value=K_CAN_GMLAN_RX_INVALID_SELECT  OutDataTypeStr=Inherit: Inherit via back propagation
  Logical Operator : Logic  Operator=OR  AllPortsSameDT=off  OutDataTypeStr=boolean
  Logical Operator1 : Logic  Operator=NOT  AllPortsSameDT=off  OutDataTypeStr=boolean
  Max : Constant  Value=255.996  OutDataTypeStr=Inherit: Inherit via back propagation
  Min : Constant  Value=0  OutDataTypeStr=Inherit: Inherit via back propagation
  Switch : Switch  Criteria=u2 > Threshold  SaturateOnIntegerOverflow=off  InputSameDT=off
  Switch1 : Switch  Criteria=u2 > Threshold  SaturateOnIntegerOverflow=off  InputSameDT=off
  Unit Delay : UnitDelay  SampleTime=-1  HasFrameUpgradeWarning=on
  can_gmlan_rx_invalid_gps_veh_speed : Outport
  can_gmlan_rx_gps_veh_speed : Outport  Port=2
  wires:
  inv_device_vnt/1 -> Logical Operator/1
  K_CAN_GMLAN_RX_INVALID_SELECT/1 -> Switch1/2
  Data Type Conversion1/1 -> can_gmlan_rx_invalid_gps_veh_speed/1
  Logical Operator/1 -> Data Type Conversion1/1, Switch/2
  K_CAN_GMLAN_RX_DEFAULT_GPS_VEH_SPEED/1 -> Switch1/3
  Switch1/1 -> Switch/1
  Switch/1 -> can_gmlan_rx_gps_veh_speed/1, Unit Delay/1
  Logical Operator1/1 -> Logical Operator/2
  Max/1 -> Interval Test Dynamic/1
  Min/1 -> Interval Test Dynamic/3
  Unit Delay/1 -> Switch1/1
  GetData/1 -> Data Type Conversion/1
  Interval Test Dynamic/1 -> Logical Operator1/1
  Data Type Conversion/1 -> Switch/3, Interval Test Dynamic/2
